simulink model "puma560withSineInput"  (R2014a)
settings: Solver=ode3  StartTime=0.0  StopTime=inf  FixedStep=0.1  RelTol=1e-3
libraries: roblocks x5, simulink x1
settings Model: ExtModeTrigMode=oneshot  ExtModeArmWhenConnect=off  ExtModeAutoUpdateStatusClock=off  Creator=pic  LastModifiedBy=Edoardo
settings DataIOCC: LimitDataPoints=off  SignalLoggingSaveFormat=ModelDataLogs  SignalLoggingName=sigsOut
settings OptimizationCC: BlockReduction=off  BooleanDataType=off  ExpressionDepthLimit=2147483647
settings DebuggingCC: SaveWithParameterizedLinksMsg=none  UnderspecifiedInitializationDetection=Classic  SignalResolutionControl=TryResolveAllWithWarning  SolverPrmCheckMsg=none  MultiTaskDSMMsg=warning  MultiTaskCondExecSysMsg=none  FcnCallInpInsideContextMsg=UseLocalSettings  StateNameClashWarn=warning
settings HardwareCC: TargetUnknown=on
settings RTWCC: IncludeERTFirstTime=on
settings GRTTargetCC: CombineOutputUpdateFcns=off  GRTInterface=on

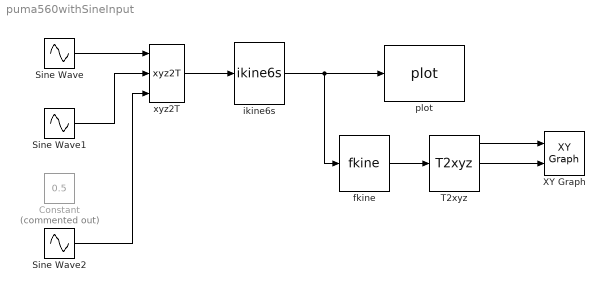
== system puma560withSineInput ==
  Constant : Constant  Commented=on  Value=0.5
  Sine Wave : Sin  Amplitude=0.5  Frequency=0.1  SampleTime=0
  Sine Wave1 : Sin  Amplitude=0.5  Frequency=0.1  Phase=pi/2  SampleTime=0
  Sine Wave2 : Sin  Amplitude=0.1  Bias=0.3  Frequency=0.2  SampleTime=0
  T2xyz : roblocks/Transform Conversion/T2xyz
  XY Graph : simulink/Sinks/XY Graph  xmin=-1  xmax=1  ymin=-1  ymax=1  st=-1
  fkine : roblocks/Kinematics/fkine  robot=p560
  ikine6s : roblocks/Kinematics/ikine6s  robot=p560  conf='luf'
  plot : roblocks/Robot Graphics/plot  robot=p560  fps=25  holdplot=on
  xyz2T : roblocks/Transform Conversion/xyz2T
  wires:
  ikine6s/1 -> plot/1, fkine/1
  fkine/1 -> T2xyz/1
  T2xyz/1 -> XY Graph/1
  T2xyz/2 -> XY Graph/2
  xyz2T/1 -> ikine6s/1
  Sine Wave/1 -> xyz2T/1
  Sine Wave1/1 -> xyz2T/2
  Sine Wave2/1 -> xyz2T/3
